simulink model "Complete_vehicle_simulation_dof14_model"  (R2024b)
settings: Solver=FixedStepAuto  StartTime=0.0  StopTime=10  FixedStep=0.001  RelTol=1e-3
values from neighbouring files (symbols this model uses):
  a = 1.8    [Complete_vehicle_simulation_dof14_model_parameters.m]
  A = 1.25    [Complete_vehicle_simulation_dof14_model_parameters.m]
  a1f = -1e-5    (= -1e-05)    [Complete_vehicle_simulation_dof14_model_parameters.m]
  a1r = -1e-5    (= -1e-05)    [Complete_vehicle_simulation_dof14_model_parameters.m]
  a2f = 0.95    [Complete_vehicle_simulation_dof14_model_parameters.m]
  a2r = 0.95    [Complete_vehicle_simulation_dof14_model_parameters.m]
  b = L-a    (= 1.7)    [Complete_vehicle_simulation_dof14_model_parameters.m]
  balance = 0.65    [Complete_vehicle_simulation_dof14_model_parameters.m]
  Bf = 0.0813    [Complete_vehicle_simulation_dof14_model_parameters.m]
  Br = 0.0925    [Complete_vehicle_simulation_dof14_model_parameters.m]
  Cd = 0.4    [Complete_vehicle_simulation_dof14_model_parameters.m]
  cdf = 1400    [Complete_vehicle_simulation_dof14_model_parameters.m]
  cdr = 1800    [Complete_vehicle_simulation_dof14_model_parameters.m]
  Cf = 1.2947    [Complete_vehicle_simulation_dof14_model_parameters.m]
  Cr = 1.2617    [Complete_vehicle_simulation_dof14_model_parameters.m]
  Cz = 1.0    (= 1)    [Complete_vehicle_simulation_dof14_model_parameters.m]
  Ef = -8.3966    [Complete_vehicle_simulation_dof14_model_parameters.m]
  enginemap = [-0.15, 0.23, 0.60, 0.68, 0.8 ... (first row only)    [Complete_vehicle_simulation_dof14_model_parameters.m]
  enginerpm = linspace (1000,15000,15)'    [Complete_vehicle_simulation_dof14_model_parameters.m]
  Er = -8.7012    [Complete_vehicle_simulation_dof14_model_parameters.m]
  g = 9.81    [Complete_vehicle_simulation_dof14_model_parameters.m]
  h = 0.2    [Complete_vehicle_simulation_dof14_model_parameters.m]
  hrcf = 0.04    [Complete_vehicle_simulation_dof14_model_parameters.m]
  hrcr = 0.06    [Complete_vehicle_simulation_dof14_model_parameters.m]
  husmf = r    (= 0.375)    [Complete_vehicle_simulation_dof14_model_parameters.m]
  husmr = r    (= 0.375)    [Complete_vehicle_simulation_dof14_model_parameters.m]
  I = 3500    [Complete_vehicle_simulation_dof14_model_parameters.m]
  igear = [23.10, 17.64, 13.86, 10.92, 8.82, 7.14, 5.88, 4.33]'    [Complete_vehicle_simulation_dof14_model_parameters.m]
  Iwheel = 0.9    [Complete_vehicle_simulation_dof14_model_parameters.m]
  Ixx = 300    [Complete_vehicle_simulation_dof14_model_parameters.m]
  Iyy = 1350    [Complete_vehicle_simulation_dof14_model_parameters.m]
  karbf = 5000    [Complete_vehicle_simulation_dof14_model_parameters.m]
  karbr = 1000    [Complete_vehicle_simulation_dof14_model_parameters.m]
  ksf = 67500    [Complete_vehicle_simulation_dof14_model_parameters.m]
  ksr = 100000    [Complete_vehicle_simulation_dof14_model_parameters.m]
  ktyre = 400000    [Complete_vehicle_simulation_dof14_model_parameters.m]
  L = 3.5    [Complete_vehicle_simulation_dof14_model_parameters.m]
  m = 850    [Complete_vehicle_simulation_dof14_model_parameters.m]
  ms = m-(musf+musr)    (= 817.5)    [Complete_vehicle_simulation_dof14_model_parameters.m]
  musf = 15.00    (= 15)    [Complete_vehicle_simulation_dof14_model_parameters.m]
  musr = 17.50    (= 17.5)    [Complete_vehicle_simulation_dof14_model_parameters.m]
  r = 0.375    [Complete_vehicle_simulation_dof14_model_parameters.m]
  rbrake = 3800    [Complete_vehicle_simulation_dof14_model_parameters.m]
  rho = 1.225    [Complete_vehicle_simulation_dof14_model_parameters.m]
  rpm_idling = 1000    [Complete_vehicle_simulation_dof14_model_parameters.m]
  rpm_limit = 15000    [Complete_vehicle_simulation_dof14_model_parameters.m]
  rpm_up = 13500    [Complete_vehicle_simulation_dof14_model_parameters.m]
  Tengmax = 250    [Complete_vehicle_simulation_dof14_model_parameters.m]
  throttlepos = [0, 0.25, 0.5, 0.75, 1]'    [Complete_vehicle_simulation_dof14_model_parameters.m]
  tr = 1.85    [Complete_vehicle_simulation_dof14_model_parameters.m]
  z0tfl = (0.5*ms*b/L+musf)*g/ktyre    (= 0.00523696339286)    [Complete_vehicle_simulation_dof14_model_parameters.m]
  z0tfr = (0.5*ms*b/L+musf)*g/ktyre    (= 0.00523696339286)    [Complete_vehicle_simulation_dof14_model_parameters.m]
  z0trl = (0.5*ms*a/L+musr)*g/ktyre    (= 0.00558469285714)    [Complete_vehicle_simulation_dof14_model_parameters.m]
  z0trr = (0.5*ms*a/L+musr)*g/ktyre    (= 0.00558469285714)    [Complete_vehicle_simulation_dof14_model_parameters.m]
libraries: aerolibconvert2 x8, simulink x1
settings Model: Creator=jayku  LastModifiedBy=jayku

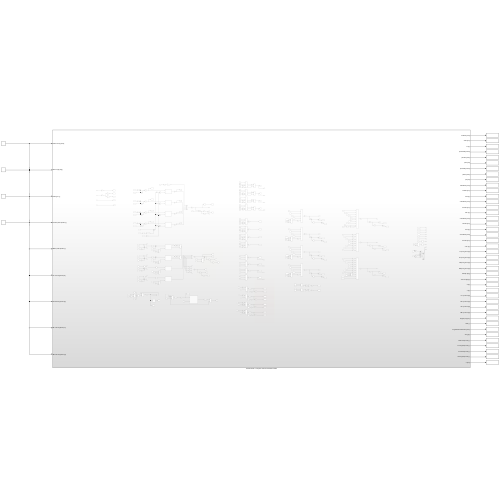
[thumbnail: Simulink's stored preview of the top-level diagram]
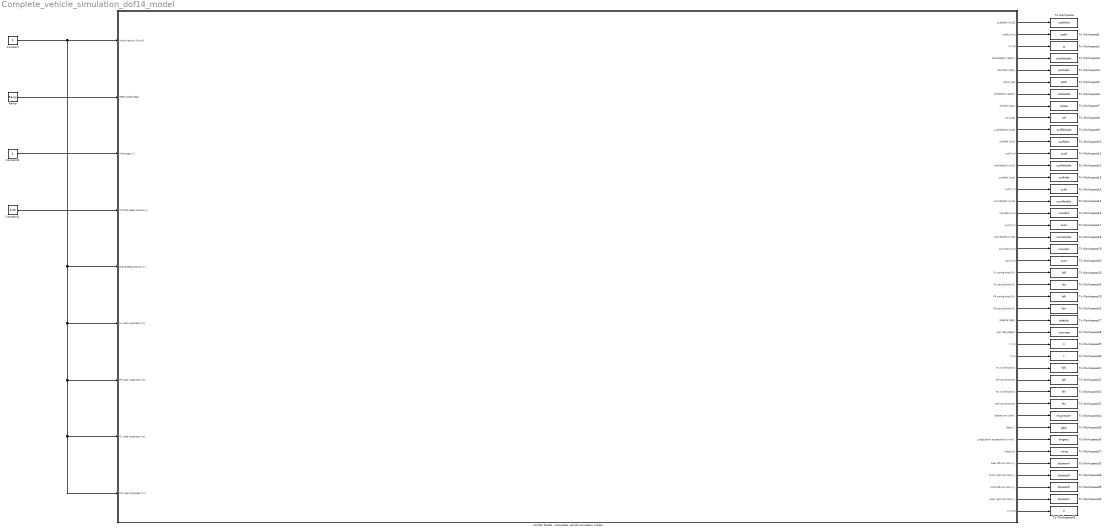
== system Complete_vehicle_simulation_dof14_model ==
  14 DoF Model - Complete vehicle simulation model : Subsystem
  Constant : Constant  Value=0
  Constant1 : Constant  Value=0.05
  Constant2 : Constant  Value=3
  Ramp : simulink/Sources/Ramp  slope=1  start=0  InitialOutput=0
  To Workspace : ToWorkspace  VariableName=zsdotdot  SaveFormat=Timeseries  SampleTime=-1
  To Workspace1 : ToWorkspace  VariableName=zsdot  SaveFormat=Timeseries  SampleTime=-1
  To Workspace10 : ToWorkspace  VariableName=zusfldot  SaveFormat=Timeseries  SampleTime=-1
  To Workspace11 : ToWorkspace  VariableName=zusfl  SaveFormat=Timeseries  SampleTime=-1
  To Workspace12 : ToWorkspace  VariableName=zusfrdotdot  SaveFormat=Timeseries  SampleTime=-1
  To Workspace13 : ToWorkspace  VariableName=zusfrdot  SaveFormat=Timeseries  SampleTime=-1
  To Workspace14 : ToWorkspace  VariableName=zusfr  SaveFormat=Timeseries  SampleTime=-1
  To Workspace15 : ToWorkspace  VariableName=zusrldotdot  SaveFormat=Timeseries  SampleTime=-1
  To Workspace16 : ToWorkspace  VariableName=zusrldot  SaveFormat=Timeseries  SampleTime=-1
  To Workspace17 : ToWorkspace  VariableName=zusrl  SaveFormat=Timeseries  SampleTime=-1
  To Workspace18 : ToWorkspace  VariableName=zusrrdotdot  SaveFormat=Timeseries  SampleTime=-1
  To Workspace19 : ToWorkspace  VariableName=zusrrdot  SaveFormat=Timeseries  SampleTime=-1
  To Workspace2 : ToWorkspace  VariableName=zs  SaveFormat=Timeseries  SampleTime=-1
  To Workspace20 : ToWorkspace  VariableName=zusrr  SaveFormat=Timeseries  SampleTime=-1
  To Workspace21 : ToWorkspace  VariableName=ftfl  SaveFormat=Timeseries  SampleTime=-1
  To Workspace22 : ToWorkspace  VariableName=ftfr  SaveFormat=Timeseries  SampleTime=-1
  To Workspace23 : ToWorkspace  VariableName=fsfl  SaveFormat=Timeseries  SampleTime=-1
  To Workspace24 : ToWorkspace  VariableName=fsrl  SaveFormat=Timeseries  SampleTime=-1
  To Workspace25 : ToWorkspace  VariableName=fsfr  SaveFormat=Timeseries  SampleTime=-1
  To Workspace26 : ToWorkspace  VariableName=fsrr  SaveFormat=Timeseries  SampleTime=-1
  To Workspace27 : ToWorkspace  VariableName=sideslip  SaveFormat=Timeseries  SampleTime=-1
  To Workspace28 : ToWorkspace  VariableName=yawrate  SaveFormat=Timeseries  SampleTime=-1
  To Workspace29 : ToWorkspace  VariableName=X  SaveFormat=Timeseries  SampleTime=-1
  To Workspace3 : ToWorkspace  VariableName=pitchdotdot  SaveFormat=Timeseries  SampleTime=-1
  To Workspace30 : ToWorkspace  VariableName=Y  SaveFormat=Timeseries  SampleTime=-1
  To Workspace31 : ToWorkspace  VariableName=ftrl  SaveFormat=Timeseries  SampleTime=-1
  To Workspace32 : ToWorkspace  VariableName=ftrr  SaveFormat=Timeseries  SampleTime=-1
  To Workspace33 : ToWorkspace  VariableName=slipratiorl  SaveFormat=Timeseries  SampleTime=-1
  To Workspace34 : ToWorkspace  VariableName=enginerpm  SaveFormat=Timeseries  SampleTime=-1
  To Workspace35 : ToWorkspace  VariableName=gear  SaveFormat=Timeseries  SampleTime=-1
  To Workspace36 : ToWorkspace  VariableName=longacc  SaveFormat=Timeseries  SampleTime=-1
  To Workspace37 : ToWorkspace  VariableName=xlong  SaveFormat=Timeseries  SampleTime=-1
  To Workspace38 : ToWorkspace  VariableName=slipratiofr  SaveFormat=Timeseries  SampleTime=-1
  To Workspace39 : ToWorkspace  VariableName=slipratiofl  SaveFormat=Timeseries  SampleTime=-1
  To Workspace4 : ToWorkspace  VariableName=pitchdot  SaveFormat=Timeseries  SampleTime=-1
  To Workspace40 : ToWorkspace  VariableName=slipratiorr  SaveFormat=Timeseries  SampleTime=-1
  To Workspace41 : ToWorkspace  VariableName=V  SaveFormat=Timeseries  SampleTime=-1
  To Workspace5 : ToWorkspace  VariableName=pitch  SaveFormat=Timeseries  SampleTime=-1
  To Workspace6 : ToWorkspace  VariableName=rolldotdot  SaveFormat=Timeseries  SampleTime=-1
  To Workspace7 : ToWorkspace  VariableName=rolldot  SaveFormat=Timeseries  SampleTime=-1
  To Workspace8 : ToWorkspace  VariableName=roll  SaveFormat=Timeseries  SampleTime=-1
  To Workspace9 : ToWorkspace  VariableName=zusfldotdot  SaveFormat=Timeseries  SampleTime=-1
  wires:
  14 DoF Model - Complete vehicle simulation model/1(zsdotdot [m/s2]) -> To Workspace/1
  14 DoF Model - Complete vehicle simulation model/2(zsdot [m/s]) -> To Workspace1/1
  14 DoF Model - Complete vehicle simulation model/3(zs [m]) -> To Workspace2/1
  14 DoF Model - Complete vehicle simulation model/4(pitchdotdot [rad/s2]) -> To Workspace3/1
  14 DoF Model - Complete vehicle simulation model/5(pitchdot [rad/s]) -> To Workspace4/1
  14 DoF Model - Complete vehicle simulation model/6(pitch [rad]) -> To Workspace5/1
  14 DoF Model - Complete vehicle simulation model/7(phidotdot [rad/s2]) -> To Workspace6/1
  14 DoF Model - Complete vehicle simulation model/8(phidot [rad/s]) -> To Workspace7/1
  14 DoF Model - Complete vehicle simulation model/9(phi [rad]) -> To Workspace8/1
  14 DoF Model - Complete vehicle simulation model/10(zusfldotdot [m/s2]) -> To Workspace9/1
  14 DoF Model - Complete vehicle simulation model/11(zusfldot [m/s]) -> To Workspace10/1
  14 DoF Model - Complete vehicle simulation model/12(zusfl [m]) -> To Workspace11/1
  14 DoF Model - Complete vehicle simulation model/13(zusfrdotdot [m/s2]) -> To Workspace12/1
  14 DoF Model - Complete vehicle simulation model/14(zusfrdot [m/s]) -> To Workspace13/1
  14 DoF Model - Complete vehicle simulation model/15(zusfr [m]) -> To Workspace14/1
  14 DoF Model - Complete vehicle simulation model/16(zusrldotdot [m/s2]) -> To Workspace15/1
  14 DoF Model - Complete vehicle simulation model/17(zusrldot [m/s]) -> To Workspace16/1
  14 DoF Model - Complete vehicle simulation model/18(zusrl [m]) -> To Workspace17/1
  14 DoF Model - Complete vehicle simulation model/19(zusrrdotdot [m/s2]) -> To Workspace18/1
  14 DoF Model - Complete vehicle simulation model/20(zusrrdot [m/s]) -> To Workspace19/1
  14 DoF Model - Complete vehicle simulation model/21(zusrr [m]) -> To Workspace20/1
  14 DoF Model - Complete vehicle simulation model/22(FL spring force [N]) -> To Workspace23/1
  14 DoF Model - Complete vehicle simulation model/23(RL spring force [N]) -> To Workspace24/1
  14 DoF Model - Complete vehicle simulation model/24(FR spring force [N]) -> To Workspace25/1
  14 DoF Model - Complete vehicle simulation model/25(RR spring force [N]) -> To Workspace26/1
  14 DoF Model - Complete vehicle simulation model/26(Sideslip [deg]) -> To Workspace27/1
  14 DoF Model - Complete vehicle simulation model/27(Yaw rate [deg/s]) -> To Workspace28/1
  14 DoF Model - Complete vehicle simulation model/28(X [m]) -> To Workspace29/1
  14 DoF Model - Complete vehicle simulation model/29(Y [m]) -> To Workspace30/1
  14 DoF Model - Complete vehicle simulation model/30(FL tyre force [N]) -> To Workspace21/1
  14 DoF Model - Complete vehicle simulation model/31(FR tyre force [N]) -> To Workspace22/1
  14 DoF Model - Complete vehicle simulation model/32(RL tyre force [N]) -> To Workspace31/1
  14 DoF Model - Complete vehicle simulation model/33(RR tyre force [N]) -> To Workspace32/1
  14 DoF Model - Complete vehicle simulation model/38(Rear left slip ratio [-]) -> To Workspace33/1
  14 DoF Model - Complete vehicle simulation model/34(Engine rpm [rpm]) -> To Workspace34/1
  14 DoF Model - Complete vehicle simulation model/35(Gear [-]) -> To Workspace35/1
  14 DoF Model - Complete vehicle simulation model/36(Longitudinal acceleration [km/h]) -> To Workspace36/1
  14 DoF Model - Complete vehicle simulation model/37(xlong [m]) -> To Workspace37/1
  14 DoF Model - Complete vehicle simulation model/39(Front right slip ratio [-]) -> To Workspace38/1
  14 DoF Model - Complete vehicle simulation model/40(Front left slip ratio [-]) -> To Workspace39/1
  14 DoF Model - Complete vehicle simulation model/41(Rear right slip ratio [-]) -> To Workspace40/1
  Constant/1 -> 14 DoF Model - Complete vehicle simulation model/8(RL road roughness [m]), 14 DoF Model - Complete vehicle simulation model/9(RR road roughness [m]), 14 DoF Model - Complete vehicle simulation model/7(FR road roughness [m]), 14 DoF Model - Complete vehicle simulation model/6(FL road roughness [m]), 14 DoF Model - Complete vehicle simulation model/5(Brake pedal position [-]), 14 DoF Model - Complete vehicle simulation model/1(Initial velocity [km/h])
  Constant1/1 -> 14 DoF Model - Complete vehicle simulation model/4(Throttle pedal position [-])
  Ramp/1 -> 14 DoF Model - Complete vehicle simulation model/2(Steer angle [deg])
  Constant2/1 -> 14 DoF Model - Complete vehicle simulation model/3(Initial gear [-])
  14 DoF Model - Complete vehicle simulation model/42(V [m/s]) -> To Workspace41/1

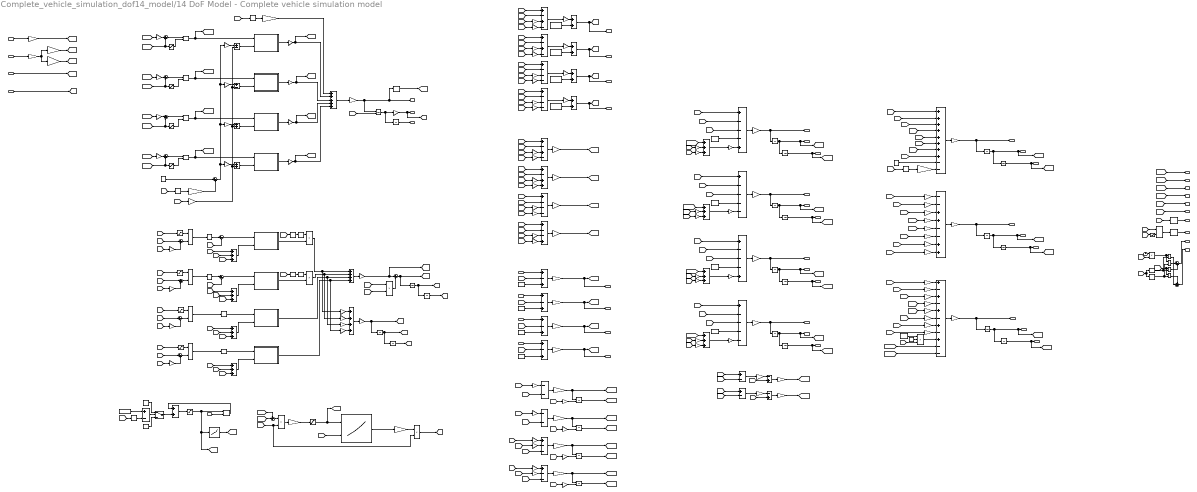
== system Complete_vehicle_simulation_dof14_model/14 DoF Model - Complete vehicle simulation model ==
  Initial velocity [km/h] : Inport
  Steer angle [deg] : Inport  Port=2
  Initial gear [-] : Inport  Port=3
  Throttle pedal position [-] : Inport  Port=4
  Brake pedal position [-] : Inport  Port=5
  FL road roughness [m] : Inport  Port=6
  FR road roughness [m] : Inport  Port=7
  RL road roughness [m] : Inport  Port=8
  RR road roughness [m] : Inport  Port=9
  1-D Lookup Table : Lookup_n-D  NumberOfTableDimensions=1  BreakpointsForDimension1=[1:8]  Table=igear  InternalRulePriority=Speed  RndMeth=Simplest
  2-D Lookup Table : Lookup_n-D  BreakpointsForDimension1=enginerpm  BreakpointsForDimension2=throttlepos  Table=enginemap  InternalRulePriority=Speed  RndMeth=Simplest
      settings: InputPortMap=u0,u1
  Add : Sum  Inputs=++++++++--
  Add1 : Sum  Inputs=--++--++
  Add{3..4,10,12,15,17,44..45} (8 alike) : Sum  Inputs=+++
  Add11 : Sum  Inputs=++++
  Add16 : Sum  Inputs=+++++
  Add18 : Sum  Inputs=--
  Add{19,33..34,40..41} (5 alike) : Sum  Inputs=+-
  Add2 : Sum  Inputs=+-+-+-+-+--
  Add20 : Sum  Inputs=+-+-
  Add{21,23,25,27,37,42..43} (7 alike) : Sum
  Add22 : Sum  Inputs=+-+-
  Add24 : Sum  Inputs=+---
  Add26 : Sum  Inputs=+---
  Add28 : Sum  Inputs=+-+-
  Add29 : Sum  Inputs=+-++
  Add30 : Sum  Inputs=+---
  Add31 : Sum  Inputs=+--+
  Add32 : Sum  Inputs=-+
  Add35 : Sum  Inputs=-+
  Add36 : Sum  Inputs=--
  Add38 : Sum  Inputs=+--
  Add39 : Sum  Inputs=+--
  Add5 : Sum  Inputs=++++
  Add{6..9} (4 alike) : Sum  Inputs=+-+
  Angle Conversion{,4..8} (6 alike) : aerolibconvert2/Angle Conversion  IU=rad  OU=deg
  Angle Conversion2 : aerolibconvert2/Angle Conversion  IU=deg  OU=rad
  Angle Conversion3 : aerolibconvert2/Angle Conversion  IU=deg  OU=rad
  Clock : Clock
  Constant : Constant  Value=ms*g
  Constant10 : Constant  Value=z0tfr
  Constant11 : Constant  Value=0.5*ms*g*a/L
  Constant12 : Constant  Value=z0trl
  Constant13 : Constant  Value=z0trr
  Constant14 : Constant  Value=m*g
  Constant15 : Constant
  Constant16 : Constant  Value=musr*g
  Constant17 : Constant  Value=rpm_up
  Constant18 : Constant  Value=0
  Constant2 : Constant  Value=hcog-hrc
  Constant20 : Constant  Value=musr*g
  Constant3 : Constant  Value=0.5*ms*g*b/L
  Constant4 : Constant  Value=musf*g
  Constant5 : Constant  Value=0.5*ms*g*b/L
  Constant6 : Constant  Value=ms
  Constant7 : Constant  Value=0.5*ms*g*a/L
  Constant8 : Constant  Value=z0tfl
  Constant9 : Constant  Value=musf*g
  Cos : Trigonometry  Operator=cos
  Cos2 : Trigonometry  Operator=cos
  Cos3 : Trigonometry  Operator=cos
  Delay : Delay  DelayLength=1  InitialConditionSource=Input port  InitialCondition=0
      settings: InputPortMap=u0,p4
  Delay1 : Delay  DelayLength=1  InitialCondition=0
  Delay3 : Delay  DelayLength=1  InitialCondition=0
  Front left : Sum  Inputs=+---+
  Front left pacejka longitudinal tyre : Subsystem
  Front right : Sum  Inputs=+----
  Front right pacejka longitudinal tyre : Subsystem
  Gain : Gain  Gain=1/ms
  Gain1 : Gain  Gain=1/Iyy
  Gain10 : Gain  Gain=1/Ixx
  Gain{80,83,97,100..103,106} (8 alike) : Gain  Gain=r
  Gain104 : Gain  Gain=Tengmax
  Gain105 : Gain  Gain=60/(2*pi)
  Gain107 : Gain  Gain=b/L
  Gain108 : Gain  Gain=a/L
  Gain109 : Gain  Gain=0.5*rho*A*Cz
  Gain{11..13,15,56,59,68,71} (8 alike) : Gain  Gain=tr/2
  Gain{93..94,110..111} (4 alike) : Gain  Gain=-1
  Gain112 : Gain  Gain=-1/m
  Gain113 : Gain  Gain=3.6
  Gain{6..9,54,57,66,69,88..90,114} (12 alike) : Gain  Gain=b
  Gain{2..5,43..45,48,51,60,63,115} (12 alike) : Gain  Gain=a
  Gain116 : Gain  Gain=1/I
  Gain{14,16..18,50,53,62,65} (8 alike) : Gain  Gain=tf/2
  Gain{19..22} (4 alike) : Gain  Gain=ktyre
  Gain23 : Gain  Gain=0.5*rho*A*Cz
  Gain24 : Gain  Gain=ms*a/L*hrcr
  Gain25 : Gain  Gain=2*musr*husmr
  Gain26 : Gain  Gain=ms*b/L*hrcf
  Gain27 : Gain  Gain=2*musf*husmf
  Gain28 : Gain  Gain=1/tf
  Gain29 : Gain  Gain=1/musf
  Gain30 : Gain  Gain=1/2
  Gain31 : Gain  Gain=1/2
  Gain32 : Gain  Gain=ms*b/L*hrcf
  Gain33 : Gain  Gain=2*musf*husmf
  Gain34 : Gain  Gain=1/tf
  Gain35 : Gain  Gain=1/musf
  Gain38 : Gain  Gain=ms*a/L*hrcr
  Gain39 : Gain  Gain=2*musr*husmr
  Gain40 : Gain  Gain=1/tr
  Gain41 : Gain  Gain=1/musr
  Gain42 : Gain  Gain=1/m
  Gain46 : Gain  Gain=1/tr
  Gain47 : Gain  Gain=1/musr
  Gain49 : Gain  Gain=ksf
  Gain52 : Gain  Gain=ksf
  Gain55 : Gain  Gain=ksr
  Gain58 : Gain  Gain=ksr
  Gain61 : Gain  Gain=cdf
  Gain64 : Gain  Gain=cdf
  Gain67 : Gain  Gain=cdr
  Gain70 : Gain  Gain=cdr
  Gain72 : Gain  Gain=1/tf
  Gain73 : Gain  Gain=karbf
  Gain74 : Gain  Gain=1/tr
  Gain75 : Gain  Gain=karbr
  Gain76 : Gain  Gain=0.5*rho*A*Cd
  Gain77 : Gain  Gain=b/L
  Gain{78,81,95,98} (4 alike) : Gain  Gain=1/Iwheel
  Gain{79,82,96,99} (4 alike) : Gain  Gain=1/r
  Gain84 : Gain  Gain=rbrake
  Gain85 : Gain  Gain=balance
  Gain86 : Gain  Gain=1/3.6
  Gain87 : Gain  Gain=(1-balance)
  Gain91 : Gain  Gain=m*h/L
  Gain92 : Gain  Gain=a/L
  Integrator{,1..13,18..19,25..27} (19 alike) : Integrator
  Integrator{20..24} (5 alike) : Integrator  InitialConditionSource=external
  Pacejka front left lateral tyre model : Subsystem
  Pacejka front right lateral tyre model : Subsystem
  Pacejka rear left lateral tyre model : Subsystem
  Pacejka rear right lateral tyre model : Subsystem
  Product : Product  Inputs=***
  Product{3..4,6..10,21} (8 alike) : Product
  Product{11..12,19..20} (4 alike) : Product  Inputs=/*
  Product{5,13,16..18} (5 alike) : Product  Inputs=*/
  Product14 : Product  Inputs=**
  Product15 : Product  Inputs=**
  Rear left : Sum  Inputs=+---+
  Rear left pacejka longitudinal tyre : Subsystem
  Rear left pacejka longitudinal tyre1 : Subsystem
  Rear right : Sum  Inputs=+----
  Saturation{1..2,5..6,8..12} (9 alike) : Saturate  UpperLimit=inf  LowerLimit=0.5
  Saturation3 : Saturate  UpperLimit=rpm_limit  LowerLimit=rpm_idling
  Saturation4 : Saturate  UpperLimit=length(igear)  LowerLimit=1
  Sin : Trigonometry
  Square : Math  Operator=square
  Square2 : Math  Operator=square
  Square3 : Math  Operator=square
  Sum10 : Sum  Inputs=|++
  Sum11 : Sum  Inputs=|++
  Sum{3,7,12,14..17,19..21} (10 alike) : Sum  Inputs=|+-
  Sum13 : Sum  Inputs=++|
  Sum18 : Sum  Inputs=|++
  Sum8 : Sum  Inputs=++|
  Switch : Switch  Criteria=u2 > Threshold  SaturateOnIntegerOverflow=off  InputSameDT=off
  zsdotdot [m/s2] : Outport
  zsdot [m/s] : Outport  Port=2
  zs [m] : Outport  Port=3
  pitchdotdot [rad/s2] : Outport  Port=4
  pitchdot [rad/s] : Outport  Port=5
  pitch [rad] : Outport  Port=6
  phidotdot [rad/s2] : Outport  Port=7
  phidot [rad/s] : Outport  Port=8
  phi [rad] : Outport  Port=9
  zusfldotdot [m/s2] : Outport  Port=10
  zusfldot [m/s] : Outport  Port=11
  zusfl [m] : Outport  Port=12
  zusfrdotdot [m/s2] : Outport  Port=13
  zusfrdot [m/s] : Outport  Port=14
  zusfr [m] : Outport  Port=15
  zusrldotdot [m/s2] : Outport  Port=16
  zusrldot [m/s] : Outport  Port=17
  zusrl [m] : Outport  Port=18
  zusrrdotdot [m/s2] : Outport  Port=19
  zusrrdot [m/s] : Outport  Port=20
  zusrr [m] : Outport  Port=21
  FL spring force [N] : Outport  Port=22
  RL spring force [N] : Outport  Port=23
  FR spring force [N] : Outport  Port=24
  RR spring force [N] : Outport  Port=25
  Sideslip [deg] : Outport  Port=26
  Yaw rate [deg/s] : Outport  Port=27
  X [m] : Outport  Port=28
  Y [m] : Outport  Port=29
  FL tyre force [N] : Outport  Port=30
  FR tyre force [N] : Outport  Port=31
  RL tyre force [N] : Outport  Port=32
  RR tyre force [N] : Outport  Port=33
  Engine rpm [rpm] : Outport  Port=34
  Gear [-] : Outport  Port=35
  Longitudinal acceleration [km/h] : Outport  Port=36
  xlong [m] : Outport  Port=37
  Rear left slip ratio [-] : Outport  Port=38
  Front right slip ratio [-] : Outport  Port=39
  Front left slip ratio [-] : Outport  Port=40
  Rear right slip ratio [-] : Outport  Port=41
  V [m/s] : Outport  Port=42
  wires:
  Integrator1/1 -> [zs], zs [m]/1  "Sprung mass vertical displacement [m]"
  Add/1 -> Gain/1
  [fsrr] -> Add/4
  [fsfl] -> Add/1
  [fsrl] -> Add/3
  Integrator/1 -> [zsdot], zsdot [m/s]/1, Integrator1/1  "Sprung mass vertical velocity [m/s]"
  [fsfr] -> Add/2
  [fdfl] -> Add/5
  [fdfr] -> Add/6
  [fdrl] -> Add/7
  [fdrr] -> Add/8
  Constant/1 -> Add/9
  [V] -> Square/1
  Gain/1 -> zsdotdot [m/s2]/1, Integrator/1  "Sprung mass vertical acceleration [m/s2]"
  [fdrl] -> Gain8/1
  [fdfl] -> Gain4/1
  Add1/1 -> Gain1/1
  Integrator3/1 -> [pitch], pitch [rad]/1  "Sprung mass pitch displacement [rad]"
  [fdrr] -> Gain9/1
  [fsfl] -> Gain2/1
  Integrator2/1 -> [pitchdot], pitchdot [rad/s]/1, Integrator3/1  "Sprung mass pitch velocity [rad/s]"
  [fsfr] -> Gain3/1
  Gain1/1 -> pitchdotdot [rad/s2]/1, Integrator2/1  "Sprung mass pitch acceleration [rad/s2]"
  [fsrl] -> Gain6/1
  [fsrr] -> Gain7/1
  [fdfr] -> Gain5/1
  Gain2/1 -> Add1/1
  Gain3/1 -> Add1/2
  Gain4/1 -> Add1/5
  Gain5/1 -> Add1/6
  Gain6/1 -> Add1/3
  Gain7/1 -> Add1/4
  Gain8/1 -> Add1/7
  Gain9/1 -> Add1/8
  Gain13/1 -> Add2/8
  Gain12/1 -> Add2/7
  Gain11/1 -> Add2/4
  Gain15/1 -> Add2/3
  [fdfr] -> Gain18/1
  [fdfl] -> Gain17/1
  [fsfr] -> Gain16/1
  [fsfl] -> Gain14/1
  [fsrr] -> Gain11/1
  [fsrl] -> Gain15/1
  Gain10/1 -> phidotdot [rad/s2]/1, Integrator4/1  "Sprung mass roll acceleration [rad/s2]"
  Integrator4/1 -> Integrator5/1, [phidot], phidot [rad/s]/1  "Sprung mass roll velocity [rad/s]"
  [fdrr] -> Gain13/1
  Integrator5/1 -> [phi], phi [rad]/1  "Sprung mass roll displacement [rad]"
  Add2/1 -> Gain10/1
  [fdrl] -> Gain12/1
  Gain14/1 -> Add2/1
  Gain16/1 -> Add2/2
  Gain17/1 -> Add2/5
  Gain18/1 -> Add2/6
  Constant4/1 -> Front left/4
  [fdfl] -> Front left/3
  [fsfl] -> Front left/2
  [ftfl] -> Front left/1
  [gammaarbf] -> Add4/1
  Gain26/1 -> Add4/2
  [latacc] -> Gain26/1
  Gain27/1 -> Add4/3
  [latacc] -> Gain27/1
  Gain28/1 -> Front left/5
  Add4/1 -> Gain28/1
  Front left/1 -> Gain29/1
  Integrator7/1 -> zusfl [m]/1, [zusfl]  "FL unsprung mass displacement [m]"
  Integrator6/1 -> zusfldot [m/s]/1, [zusfldot], Integrator7/1  "FL unsprung mass velocity [m/s]"
  Gain29/1 -> Integrator6/1, zusfldotdot [m/s2]/1  "FL unsprung mass acceleration [m/s2]"
  Gain35/1 -> zusfrdotdot [m/s2]/1, Integrator8/1  "FR unsprung mass acceleration [m/s2]"
  Integrator8/1 -> Integrator9/1, [zusfrdot], zusfrdot [m/s]/1  "FR unsprung mass velocity [m/s]"
  Integrator9/1 -> [zusfr], zusfr [m]/1  "FR unsprung mass displacement [m]"
  Front right/1 -> Gain35/1
  Add10/1 -> Gain34/1
  Gain34/1 -> Front right/5
  Gain33/1 -> Add10/3
  Gain32/1 -> Add10/2
  [gammaarbf] -> Add10/1
  [ftfr] -> Front right/1
  [fsfr] -> Front right/2
  [fdfr] -> Front right/3
  Constant9/1 -> Front right/4
  Constant16/1 -> Rear left/4
  [fdrl] -> Rear left/3
  [fsrl] -> Rear left/2
  [ftrl] -> Rear left/1
  [gammaarbr] -> Add12/1
  Gain38/1 -> Add12/2
  Gain39/1 -> Add12/3
  Gain40/1 -> Rear left/5
  Add12/1 -> Gain40/1
  Rear left/1 -> Gain41/1
  Integrator11/1 -> zusrl [m]/1, [zusrl]  "RL unsprung mass displacement [m]"
  Integrator10/1 -> zusrldot [m/s]/1, [zusrldot], Integrator11/1  "RL unsprung mass velocity [m/s]"
  Gain41/1 -> Integrator10/1, zusrldotdot [m/s2]/1  "RL unsprung mass acceleration [m/s2]"
  Gain47/1 -> zusrrdotdot [m/s2]/1, Integrator12/1  "RR unsprung mass acceleration [m/s2]"
  Integrator12/1 -> Integrator13/1, [zusrrdot], zusrrdot [m/s]/1  "RR unsprung mass velocity [m/s]"
  Integrator13/1 -> [zusrr], zusrr [m]/1  "RR unsprung mass displacement [m]"
  Rear right/1 -> Gain47/1
  Add3/1 -> Gain46/1
  Gain46/1 -> Rear right/5
  [gammaarbr] -> Add3/1
  [ftrr] -> Rear right/1
  [fsrr] -> Rear right/2
  [fdrr] -> Rear right/3
  Constant20/1 -> Rear right/4
  Add21/1 -> FL spring force [N]/1, [fsfl]  "FL spring force [N]"
  Gain48/1 -> Add20/3
  Gain49/1 -> Add21/1
  [zs] -> Add20/2
  [zusfl] -> Add20/1
  Add20/1 -> Gain49/1
  [pitch] -> Gain48/1
  Constant3/1 -> Add21/2
  Gain50/1 -> Add20/4
  [phi] -> Gain50/1
  [phi] -> Gain53/1
  Gain53/1 -> Add22/4
  Constant5/1 -> Add23/2
  [pitch] -> Gain51/1
  Add22/1 -> Gain52/1
  [zusfr] -> Add22/1
  [zs] -> Add22/2
  Gain52/1 -> Add23/1
  Gain51/1 -> Add22/3
  Add23/1 -> FR spring force [N]/1, [fsfr]  "FR spring force [N]"
  Add25/1 -> RL spring force [N]/1, [fsrl]  "RL spring force [N]"
  Gain54/1 -> Add24/3
  Gain55/1 -> Add25/1
  [zs] -> Add24/2
  [zusrl] -> Add24/1
  Add24/1 -> Gain55/1
  [pitch] -> Gain54/1
  Constant7/1 -> Add25/2
  Gain56/1 -> Add24/4
  [phi] -> Gain56/1
  [phi] -> Gain59/1
  Gain59/1 -> Add26/4
  Constant11/1 -> Add27/2
  [pitch] -> Gain57/1
  Add26/1 -> Gain58/1
  [zusrr] -> Add26/1
  [zs] -> Add26/2
  Gain58/1 -> Add27/1
  Gain57/1 -> Add26/3
  Add27/1 -> RR spring force [N]/1, [fsrr]  "RR spring force [N]"
  Gain60/1 -> Add28/3
  [zsdot] -> Add28/2
  [zusfldot] -> Add28/1
  Add28/1 -> Gain61/1
  Gain61/1 -> [fdfl]  "FL damper force [N]"
  [pitchdot] -> Gain60/1
  [phidot] -> Gain62/1
  Gain62/1 -> Add28/4
  Gain65/1 -> Add29/4
  [phidot] -> Gain65/1
  [pitchdot] -> Gain63/1
  Gain64/1 -> [fdfr]  "FR damper force [N]"
  Add29/1 -> Gain64/1
  [zusfrdot] -> Add29/1
  [zsdot] -> Add29/2
  Gain63/1 -> Add29/3
  Gain66/1 -> Add30/3
  [zsdot] -> Add30/2
  [zusrldot] -> Add30/1
  Add30/1 -> Gain67/1
  Gain67/1 -> [fdrl]  "RL damper force [N]"
  [pitchdot] -> Gain66/1
  [phidot] -> Gain68/1
  Gain68/1 -> Add30/4
  Gain71/1 -> Add31/4
  [phidot] -> Gain71/1
  [pitchdot] -> Gain69/1
  Gain70/1 -> [fdrr]  "RR damper force [N]"
  Add31/1 -> Gain70/1
  [zusrrdot] -> Add31/1
  [zsdot] -> Add31/2
  Gain69/1 -> Add31/3
  Add33/1 -> Gain72/1
  [phi] -> Add32/2
  Gain72/1 -> Add32/1
  [zusfl] -> Add33/1
  Add32/1 -> Gain73/1
  [zusfr] -> Add33/2
  Gain73/1 -> [gammaarbf]  "Anti roll bar front"
  [phi] -> Add35/2
  Gain74/1 -> Add35/1
  Add34/1 -> Gain74/1
  [zusrl] -> Add34/1
  Add35/1 -> Gain75/1
  [zusrr] -> Add34/2
  Gain75/1 -> [gammaarbr]  "Anti roll bar rear"
  Gain24/1 -> Add3/2
  Gain25/1 -> Add3/3
  [latacc] -> Gain24/1
  [latacc] -> Gain25/1
  [latacc] -> Gain32/1
  [latacc] -> Gain33/1
  [latacc] -> Gain38/1
  [latacc] -> Gain39/1
  [gammaarbf] -> Add2/10
  [gammaarbr] -> Add2/11
  Constant2/1 -> Product/1
  Constant6/1 -> Product/2
  [latacc] -> Product/3
  Product/1 -> Add2/9
  Constant8/1 -> Add6/3
  FL road roughness [m]/1 -> Add6/1
  Add6/1 -> Gain19/1
  Gain19/1 -> FL tyre force [N]/1, [ftfl]  "FL tyre force [N]"
  [zusfl] -> Add6/2
  [zusfr] -> Add7/2
  Gain20/1 -> FR tyre force [N]/1, [ftfr]  "FR tyre force [N]"
  Add7/1 -> Gain20/1
  FR road roughness [m]/1 -> Add7/1
  Constant10/1 -> Add7/3
  Constant12/1 -> Add8/3
  RL road roughness [m]/1 -> Add8/1
  Add8/1 -> Gain21/1
  Gain21/1 -> RL tyre force [N]/1, [ftrl]  "RL tyre force [N]"
  [zusrl] -> Add8/2
  [zusrr] -> Add9/2
  Gain22/1 -> [ftrr], RR tyre force [N]/1  "RR tyre force [N]"
  Add9/1 -> Gain22/1
  RR road roughness [m]/1 -> Add9/1
  Constant13/1 -> Add9/3
  Gain23/1 -> Add/10
  Square/1 -> Gain23/1
  [V] -> Product6/2
  [psi] -> Cos/1, Sin/1
  Sum8/1 -> Y [m]/1
  Product5/1 -> Angle Conversion4/1
  Sin/1 -> Product9/2, Product7/2
  [y] -> Product10/1, Product9/1
  Product9/1 -> Sum7/2
  Steer angle [deg]/1 -> [delta]
  Clock/1 -> Product6/1
  Product6/1 -> Product8/1, Product7/1
  [V] -> Saturation2/1
  Cos/1 -> Product10/2, Product8/2
  Product8/1 -> Sum7/1
  Angle Conversion/1 -> Yaw rate [deg/s]/1
  Product10/1 -> Sum8/1
  [ydot] -> Product5/1
  [r] -> Angle Conversion/1
  Angle Conversion4/1 -> Sideslip [deg]/1
  Sum7/1 -> X [m]/1
  Saturation2/1 -> Product5/2
  Gain86/1 -> [V0]
  Gain85/1 -> [TBf]
  [Slipratiorr] -> Rear right slip ratio [-]/1
  [Slipratiorl] -> Rear left slip ratio [-]/1
  Gain87/1 -> [TBr]
  Initial velocity [km/h]/1 -> Gain86/1
  Brake pedal position [-]/1 -> Gain84/1
  Gain84/1 -> Gain87/1, Gain85/1
  [rpm] -> Delay1/1
  Gain104/1 -> Product14/1
  Product15/1 -> Gain105/1
  Initial gear [-]/1 -> Delay/2
  Add37/1 -> Saturation4/1
  Product14/1 -> [TD]  "Driving torque [Nm]"
  [gear] -> Gear [-]/1
  Constant17/1 -> Add19/1
  Switch/1 -> Add37/2
  Add19/1 -> Switch/2
  Throttle pedal position [-]/1 -> [throttle]
  1-D Lookup Table/1 -> [igear]
  Delay1/1 -> Add19/2
  Saturation3/1 -> [rpm], 2-D Lookup Table/1  "Engine rpm"
  Saturation4/1 -> Delay/1, 1-D Lookup Table/1, [gear]  "Engine rpm"
  2-D Lookup Table/1 -> Gain104/1  "Normalized engine torque [Nm]"
  Constant15/1 -> Switch/3
  [throttle] -> 2-D Lookup Table/2
  Delay/1 -> Add37/1
  [igear] -> Product15/2, Product14/2
  Gain105/1 -> Saturation3/1
  Constant18/1 -> Switch/1
  [rpm] -> Engine rpm [rpm]/1
  [fxfl] -> Gain80/1
  Gain79/1 -> Integrator20/2
  Integrator20/1 -> [omegafl]  "Front left rotational speed [rad/s]"
  Add18/1 -> Gain78/1
  Gain78/1 -> Integrator20/1, [omegadotfl]  "Front left rotational acceleration [rad/s2]"
  [TBf] -> Add18/2
  [V0] -> Gain79/1
  Gain80/1 -> Add18/1
  Gain83/1 -> Add36/1
  [V0] -> Gain82/1
  [TBf] -> Add36/2
  Gain81/1 -> Integrator21/1, [omegadotfr]  "Front right rotational acceleration [rad/s2]"
  Add36/1 -> Gain81/1
  Integrator21/1 -> [omegafr]  "Front right rotational speed [rad/s]"
  Gain82/1 -> Integrator21/2
  [fxfr] -> Gain83/1
  [fxrl] -> Gain97/1
  Gain96/1 -> Integrator22/2
  Integrator22/1 -> [omegarl]  "Rear left rotational speed [rad/s]"
  Add38/1 -> Gain95/1
  [TD] -> Gain30/1
  Gain95/1 -> Integrator22/1, [omegadotrl]  "Rear left rotational acceleration [rad/s2]"
  [TBr] -> Add38/3
  [V0] -> Gain96/1
  Gain97/1 -> Add38/2
  Gain100/1 -> Add39/2
  [V0] -> Gain99/1
  [TBr] -> Add39/3
  Gain98/1 -> Integrator23/1, [omegadotrr]  "Rear right rotational acceleration [rad/s2]"
  [TD] -> Gain31/1
  Add39/1 -> Gain98/1
  Integrator23/1 -> [omegarr]  "Rear right rotational speed [rad/s]"
  Gain99/1 -> Integrator23/2
  [fxrr] -> Gain100/1
  Sum13/1 -> Product15/1
  [omegarl] -> Sum13/1
  [omegarr] -> Sum13/2
  [V] -> Saturation1/1, Sum14/2
  [omegafl] -> Gain101/1
  Gain101/1 -> Sum14/1
  Product13/1 -> Front left pacejka longitudinal tyre/1(Slip ratio [-]), [Slipratiofl]  "Front slip ratio [-]"
  Sum14/1 -> Product13/1
  Sum15/1 -> Product16/1
  Product16/1 -> Front right pacejka longitudinal tyre/1(Slip ratio [-]), [Slipratiofr]  "Front slip ratio [-]"
  [V] -> Saturation8/1, Sum15/2
  Gain102/1 -> Sum15/1
  [omegafr] -> Gain102/1
  Saturation8/1 -> Product16/2
  Saturation9/1 -> Product17/2
  [omegarl] -> Gain103/1
  Gain103/1 -> Sum16/1
  [V] -> Sum16/2, Saturation9/1
  Product17/1 -> Rear left pacejka longitudinal tyre/1(Slip ratio [-]), [Slipratiorl]  "Front slip ratio [-]"
  Sum16/1 -> Product17/1
  Sum17/1 -> Product18/1
  Product18/1 -> Rear left pacejka longitudinal tyre1/1(Slip ratio [-]), [Slipratiorr]  "Front slip ratio [-]"
  [V] -> Sum17/2, Saturation10/1
  Gain106/1 -> Sum17/1
  [omegarr] -> Gain106/1
  Saturation10/1 -> Product18/2
  Add40/1 -> Front left pacejka longitudinal tyre/2(Vertical force [N])
  Add41/1 -> Front right pacejka longitudinal tyre/2(Vertical force [N])
  Add42/1 -> Rear left pacejka longitudinal tyre/2(Vertical force [N])
  Add43/1 -> Rear left pacejka longitudinal tyre1/2(Vertical force [N])
  [longacc] -> Gain91/1
  Gain91/1 -> Add43/2, Add42/2, Add41/2, Add40/2  "Load transfer [N]"
  Gain77/1 -> Add40/1
  Gain107/1 -> Add41/1
  Gain92/1 -> Add42/1
  Gain108/1 -> Add43/1
  Square3/1 -> Gain109/1
  [V] -> Square3/1
  Gain109/1 -> Sum10/2  "Downforce [N]"
  Constant14/1 -> Sum10/1
  Sum10/1 -> Gain108/1, Gain92/1, Gain107/1, Gain77/1
  Square2/1 -> Gain76/1
  [V] -> Square2/1
  Gain76/1 -> Add16/1  "Drag force [N]"
  Front left pacejka longitudinal tyre/1(Longitudinal force [N]) -> Gain93/1
  Front right pacejka longitudinal tyre/1(Longitudinal force [N]) -> Gain94/1
  Rear left pacejka longitudinal tyre/1(Longitudinal force [N]) -> Gain110/1
  Rear left pacejka longitudinal tyre1/1(Longitudinal force [N]) -> Gain111/1
  Gain93/1 -> [fxfl], Add16/2  "Front left tyre longitudinal force [N]"
  Gain94/1 -> [fxfr], Add16/3  "Front right tyre longitudinal force [N]"
  Gain110/1 -> [fxrl], Add16/4  "Rear left tyre longitudinal force [N]"
  Gain111/1 -> [fxrr], Add16/5  "Rear right tyre longitudinal force [N]"
  Delay3/1 -> [longacc]
  Integrator24/1 -> Gain113/1, Integrator25/1
  Add16/1 -> Gain112/1
  Integrator25/1 -> xlong [m]/1
  Gain112/1 -> Longitudinal acceleration [km/h]/1, Delay3/1, Integrator24/1
  [V0] -> Integrator24/2
  [Slipratiofr] -> Front right slip ratio [-]/1
  [Slipratiofl] -> Front left slip ratio [-]/1
  Saturation5/1 -> Product11/1
  [V] -> Saturation5/1
  Angle Conversion5/1 -> Sum12/1
  [delta] -> Sum12/2
  Product11/1 -> Angle Conversion5/1
  [ydot] -> Sum11/1
  Sum11/1 -> Product11/2
  Gain44/1 -> Sum11/2
  [r] -> Gain44/1
  Sum12/1 -> Pacejka front left lateral tyre model/1(Side slip angle [deg])  "Front left tyre sideslip angle [deg]"
  [r] -> Gain45/1
  Gain45/1 -> Sum18/2
  Sum18/1 -> Product12/2
  [ydot] -> Sum18/1
  Product12/1 -> Angle Conversion6/1
  [delta] -> Sum19/2
  Angle Conversion6/1 -> Sum19/1
  [V] -> Saturation6/1
  Saturation6/1 -> Product12/1
  Sum19/1 -> Pacejka front right lateral tyre model/1(Side slip angle [deg])  "Front right tyre sideslip angle [deg]"
  Saturation11/1 -> Product19/1
  Gain88/1 -> Sum20/2
  [r] -> Gain88/1
  Sum20/1 -> Product19/2
  Product19/1 -> Angle Conversion7/1
  [V] -> Saturation11/1
  [ydot] -> Sum20/1
  Angle Conversion7/1 -> Pacejka rear left lateral tyre model/1(Side slip angle [deg])  "Rear left tyre sideslip angle [deg]"
  Angle Conversion8/1 -> Pacejka rear right lateral tyre model/1(Side slip angle [deg])  "Rear right tyre sideslip angle [deg]"
  [ydot] -> Sum21/1
  [V] -> Saturation12/1
  Product20/1 -> Angle Conversion8/1
  Sum21/1 -> Product20/2
  [r] -> Gain89/1
  Gain89/1 -> Sum21/2
  Saturation12/1 -> Product20/1
  [fsfl] -> Add15/1
  [fdfl] -> Add15/2
  [ftfl] -> Add15/3
  Add15/1 -> Pacejka front left lateral tyre model/2(Vertical force [N])  "FL vertical force [N]"
  Add17/1 -> Pacejka front right lateral tyre model/2(Vertical force [N])  "FR vertical force [N]"
  [ftfr] -> Add17/3
  [fdfr] -> Add17/2
  [fsfr] -> Add17/1
  [fsrl] -> Add44/1
  [fdrl] -> Add44/2
  [ftrl] -> Add44/3
  Add44/1 -> Pacejka rear left lateral tyre model/2(Vertical force [N])  "RL vertical force [N]"
  Add45/1 -> Pacejka rear right lateral tyre model/2(Vertical force [N])  "RR vertical force [N]"
  [ftrr] -> Add45/3
  [fdrr] -> Add45/2
  [fsrr] -> Add45/1
  Angle Conversion2/1 -> Cos2/1
  Cos2/1 -> Product3/1
  [delta] -> Angle Conversion2/1
  Pacejka front left lateral tyre model/1(Lateral force [N]) -> Product3/2  "Front left tyre lateral force [N]"
  Pacejka front right lateral tyre model/1(Lateral force [N]) -> Product4/2  "Front right tyre lateral force [N]"
  [delta] -> Angle Conversion3/1
  Cos3/1 -> Product4/1
  Angle Conversion3/1 -> Cos3/1
  Pacejka rear right lateral tyre model/1(Lateral force [N]) -> Gain114/1, Add5/4  "Rear right tyre lateral force [N]"
  [V] -> Product21/1
  [r] -> Product21/2
  Integrator19/1 -> [y]
  Sum3/1 -> [ydotdot], Integrator18/1
  Add5/1 -> Gain42/1
  Gain42/1 -> Sum3/1, [latacc]  "Lateral acceleration [m/s^2]"
  Product21/1 -> Sum3/2
  Integrator18/1 -> [ydot], Integrator19/1
  Gain90/1 -> Add11/3
  Gain43/1 -> Add11/1
  Gain115/1 -> Add11/2
  Gain114/1 -> Add11/4
  Gain116/1 -> Integrator26/1, [rdot]  "Yaw acceleration [rad/s^2]"
  Integrator26/1 -> Integrator27/1, [r]  "Yaw rate [rad/s]"
  Integrator27/1 -> [psi]
  Add11/1 -> Gain116/1
  Product3/1 -> Gain43/1, Add5/1
  Product4/1 -> Gain115/1, Add5/2
  Pacejka rear left lateral tyre model/1(Lateral force [N]) -> Gain90/1, Add5/3  "Rear left tyre lateral force [N]"
  Gain30/1 -> Add38/1
  Gain31/1 -> Add39/1
  Saturation1/1 -> Product13/2
  Gain113/1 -> [V], V [m/s]/1
  Product7/1 -> Sum8/2

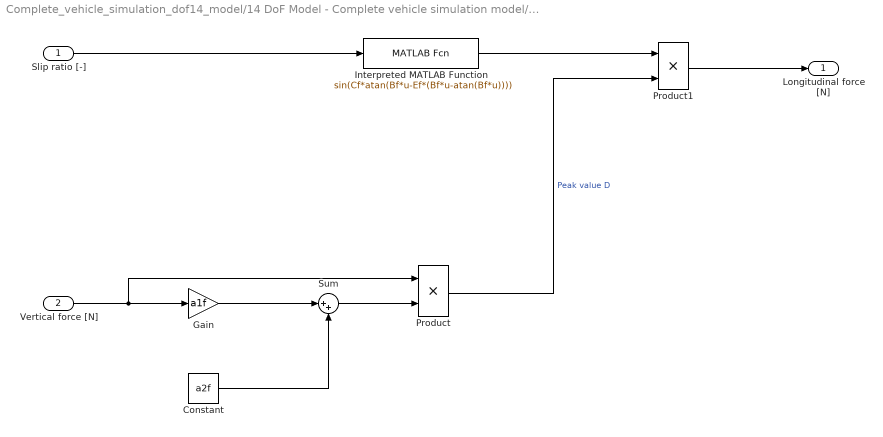
== system Complete_vehicle_simulation_dof14_model/14 DoF Model - Complete vehicle simulation model/Front left pacejka longitudinal tyre ==
  Slip ratio [-] : Inport
  Vertical force [N] : Inport  Port=2
  Constant : Constant  Value=a2f
  Gain : Gain  Gain=a1f
  Interpreted MATLAB Function : MATLABFcn  MATLABFcn=sin(Cf*atan(Bf*u-Ef*(Bf*u-atan(Bf*u))))
  Product : Product
  Product1 : Product
  Sum : Sum  Inputs=|++
  Longitudinal force [N] : Outport
  wires:
  Product1/1 -> Longitudinal force [N]/1
  Interpreted MATLAB Function/1 -> Product1/1
  Product/1 -> Product1/2  "Peak value D"
  Sum/1 -> Product/2
  Constant/1 -> Sum/2
  Gain/1 -> Sum/1
  Vertical force [N]/1 -> Gain/1, Product/1
  Slip ratio [-]/1 -> Interpreted MATLAB Function/1

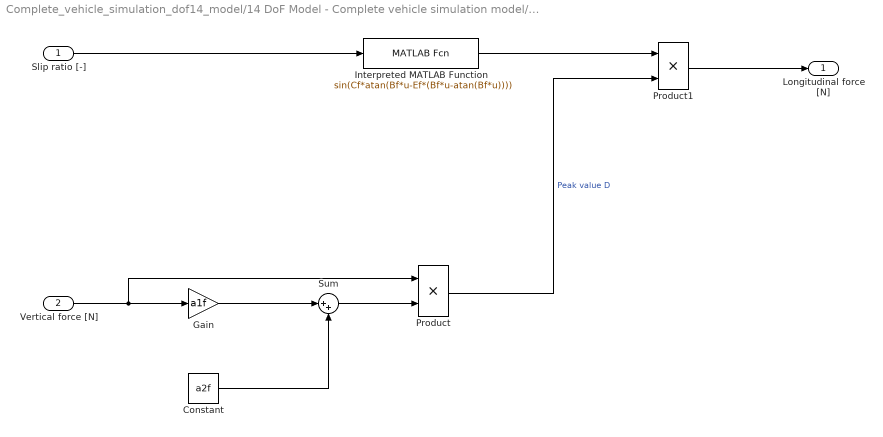
== system Complete_vehicle_simulation_dof14_model/14 DoF Model - Complete vehicle simulation model/Front right pacejka longitudinal tyre ==
  Slip ratio [-] : Inport
  Vertical force [N] : Inport  Port=2
  Constant : Constant  Value=a2f
  Gain : Gain  Gain=a1f
  Interpreted MATLAB Function : MATLABFcn  MATLABFcn=sin(Cf*atan(Bf*u-Ef*(Bf*u-atan(Bf*u))))
  Product : Product
  Product1 : Product
  Sum : Sum  Inputs=|++
  Longitudinal force [N] : Outport
  wires:
  Slip ratio [-]/1 -> Interpreted MATLAB Function/1
  Vertical force [N]/1 -> Product/1, Gain/1
  Gain/1 -> Sum/1
  Constant/1 -> Sum/2
  Sum/1 -> Product/2
  Product/1 -> Product1/2  "Peak value D"
  Interpreted MATLAB Function/1 -> Product1/1
  Product1/1 -> Longitudinal force [N]/1

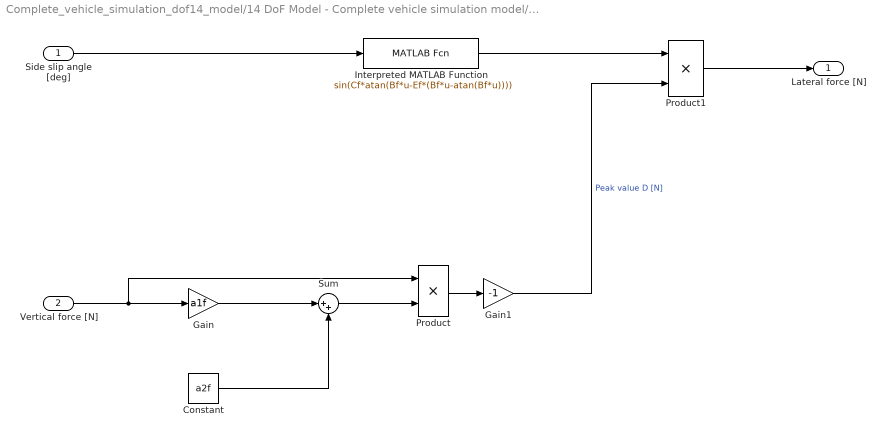
== system Complete_vehicle_simulation_dof14_model/14 DoF Model - Complete vehicle simulation model/Pacejka front left lateral tyre model ==
  Side slip angle [deg] : Inport
  Vertical force [N] : Inport  Port=2
  Constant : Constant  Value=a2f
  Gain : Gain  Gain=a1f
  Gain1 : Gain  Gain=-1
  Interpreted MATLAB Function : MATLABFcn  MATLABFcn=sin(Cf*atan(Bf*u-Ef*(Bf*u-atan(Bf*u))))
  Product : Product
  Product1 : Product
  Sum : Sum  Inputs=|++
  Lateral force [N] : Outport
  wires:
  Product1/1 -> Lateral force [N]/1
  Interpreted MATLAB Function/1 -> Product1/1
  Gain1/1 -> Product1/2  "Peak value D [N]"
  Product/1 -> Gain1/1
  Sum/1 -> Product/2
  Constant/1 -> Sum/2
  Gain/1 -> Sum/1
  Vertical force [N]/1 -> Gain/1, Product/1
  Side slip angle [deg]/1 -> Interpreted MATLAB Function/1

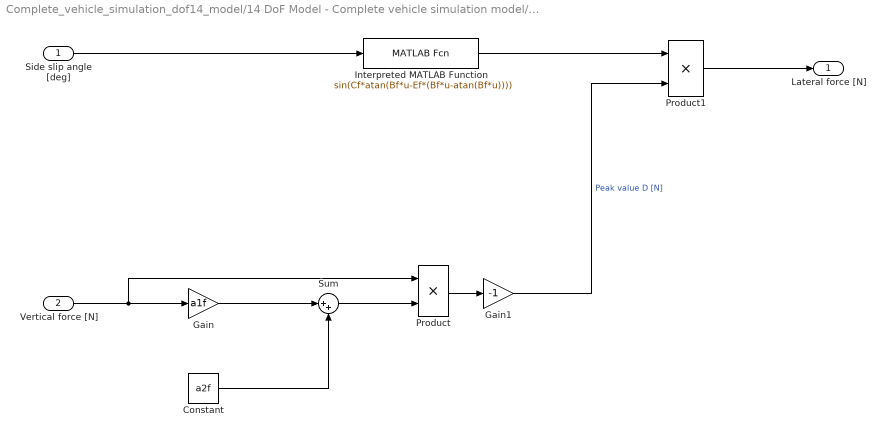
== system Complete_vehicle_simulation_dof14_model/14 DoF Model - Complete vehicle simulation model/Pacejka front right lateral tyre model ==
  Side slip angle [deg] : Inport
  Vertical force [N] : Inport  Port=2
  Constant : Constant  Value=a2f
  Gain : Gain  Gain=a1f
  Gain1 : Gain  Gain=-1
  Interpreted MATLAB Function : MATLABFcn  MATLABFcn=sin(Cf*atan(Bf*u-Ef*(Bf*u-atan(Bf*u))))
  Product : Product
  Product1 : Product
  Sum : Sum  Inputs=|++
  Lateral force [N] : Outport
  wires:
  Product1/1 -> Lateral force [N]/1
  Interpreted MATLAB Function/1 -> Product1/1
  Gain1/1 -> Product1/2  "Peak value D [N]"
  Product/1 -> Gain1/1
  Sum/1 -> Product/2
  Constant/1 -> Sum/2
  Gain/1 -> Sum/1
  Vertical force [N]/1 -> Gain/1, Product/1
  Side slip angle [deg]/1 -> Interpreted MATLAB Function/1

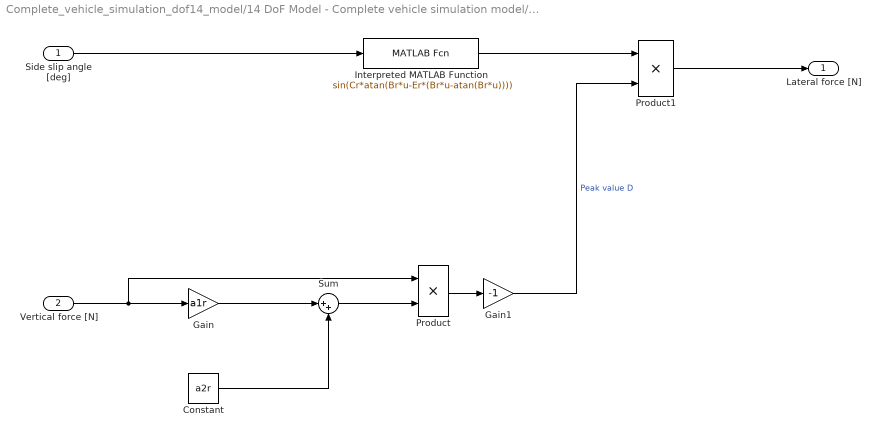
== system Complete_vehicle_simulation_dof14_model/14 DoF Model - Complete vehicle simulation model/Pacejka rear left lateral tyre model ==
  Side slip angle [deg] : Inport
  Vertical force [N] : Inport  Port=2
  Constant : Constant  Value=a2r
  Gain : Gain  Gain=a1r
  Gain1 : Gain  Gain=-1
  Interpreted MATLAB Function : MATLABFcn  MATLABFcn=sin(Cr*atan(Br*u-Er*(Br*u-atan(Br*u))))
  Product : Product
  Product1 : Product
  Sum : Sum  Inputs=|++
  Lateral force [N] : Outport
  wires:
  Product1/1 -> Lateral force [N]/1
  Interpreted MATLAB Function/1 -> Product1/1
  Gain1/1 -> Product1/2  "Peak value D"
  Product/1 -> Gain1/1
  Sum/1 -> Product/2
  Constant/1 -> Sum/2
  Gain/1 -> Sum/1
  Vertical force [N]/1 -> Gain/1, Product/1
  Side slip angle [deg]/1 -> Interpreted MATLAB Function/1

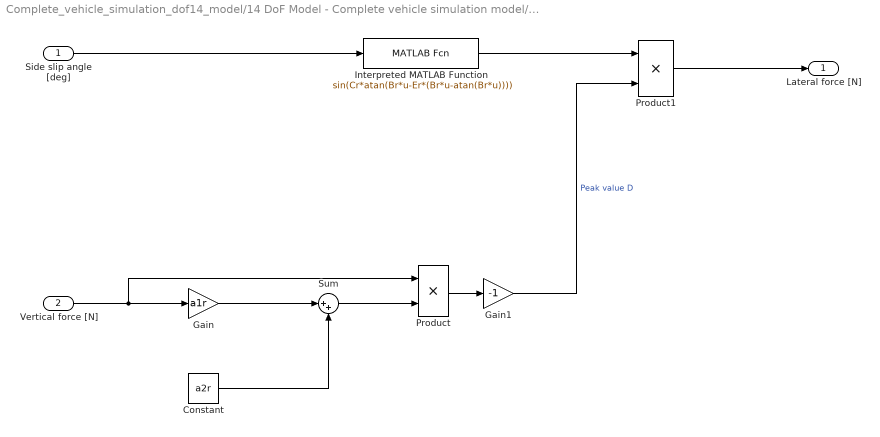
== system Complete_vehicle_simulation_dof14_model/14 DoF Model - Complete vehicle simulation model/Pacejka rear right lateral tyre model ==
  Side slip angle [deg] : Inport
  Vertical force [N] : Inport  Port=2
  Constant : Constant  Value=a2r
  Gain : Gain  Gain=a1r
  Gain1 : Gain  Gain=-1
  Interpreted MATLAB Function : MATLABFcn  MATLABFcn=sin(Cr*atan(Br*u-Er*(Br*u-atan(Br*u))))
  Product : Product
  Product1 : Product
  Sum : Sum  Inputs=|++
  Lateral force [N] : Outport
  wires:
  Product1/1 -> Lateral force [N]/1
  Interpreted MATLAB Function/1 -> Product1/1
  Gain1/1 -> Product1/2  "Peak value D"
  Product/1 -> Gain1/1
  Sum/1 -> Product/2
  Constant/1 -> Sum/2
  Gain/1 -> Sum/1
  Vertical force [N]/1 -> Gain/1, Product/1
  Side slip angle [deg]/1 -> Interpreted MATLAB Function/1

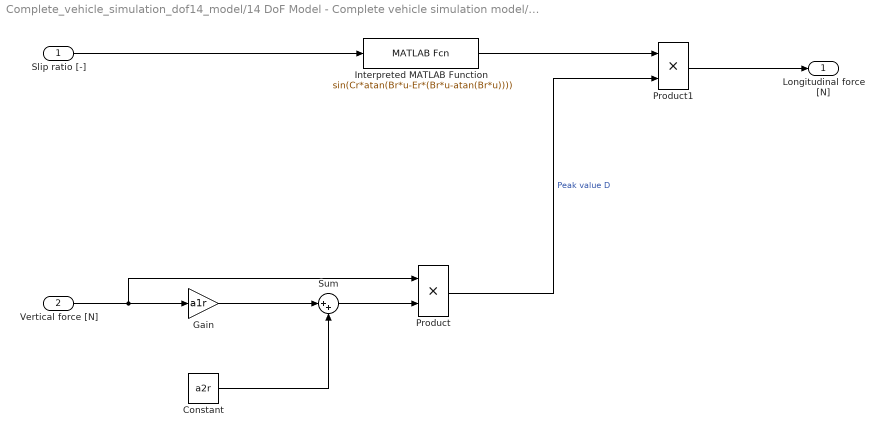
== system Complete_vehicle_simulation_dof14_model/14 DoF Model - Complete vehicle simulation model/Rear left pacejka longitudinal tyre ==
  Slip ratio [-] : Inport
  Vertical force [N] : Inport  Port=2
  Constant : Constant  Value=a2r
  Gain : Gain  Gain=a1r
  Interpreted MATLAB Function : MATLABFcn  MATLABFcn=sin(Cr*atan(Br*u-Er*(Br*u-atan(Br*u))))
  Product : Product
  Product1 : Product
  Sum : Sum  Inputs=|++
  Longitudinal force [N] : Outport
  wires:
  Product1/1 -> Longitudinal force [N]/1
  Interpreted MATLAB Function/1 -> Product1/1
  Product/1 -> Product1/2  "Peak value D"
  Sum/1 -> Product/2
  Constant/1 -> Sum/2
  Gain/1 -> Sum/1
  Vertical force [N]/1 -> Gain/1, Product/1
  Slip ratio [-]/1 -> Interpreted MATLAB Function/1

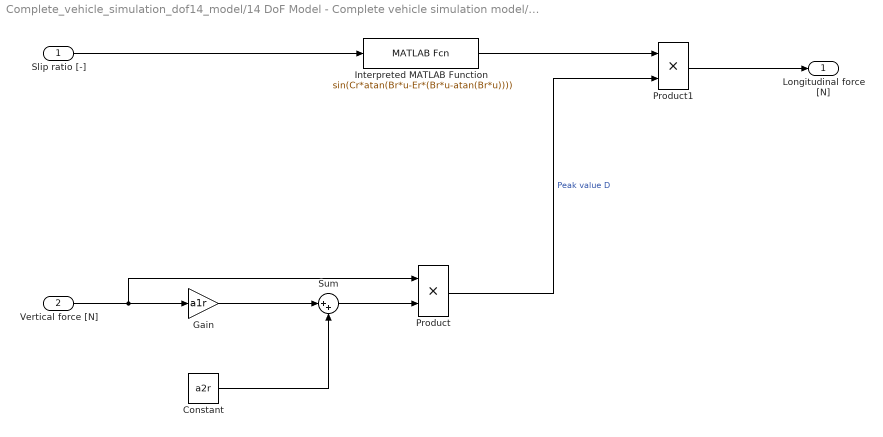
== system Complete_vehicle_simulation_dof14_model/14 DoF Model - Complete vehicle simulation model/Rear left pacejka longitudinal tyre1 ==
  Slip ratio [-] : Inport
  Vertical force [N] : Inport  Port=2
  Constant : Constant  Value=a2r
  Gain : Gain  Gain=a1r
  Interpreted MATLAB Function : MATLABFcn  MATLABFcn=sin(Cr*atan(Br*u-Er*(Br*u-atan(Br*u))))
  Product : Product
  Product1 : Product
  Sum : Sum  Inputs=|++
  Longitudinal force [N] : Outport
  wires:
  Slip ratio [-]/1 -> Interpreted MATLAB Function/1
  Vertical force [N]/1 -> Product/1, Gain/1
  Gain/1 -> Sum/1
  Constant/1 -> Sum/2
  Sum/1 -> Product/2
  Product/1 -> Product1/2  "Peak value D"
  Interpreted MATLAB Function/1 -> Product1/1
  Product1/1 -> Longitudinal force [N]/1
